simulink model "sin_osc_ver1"  (R2020a)
settings: Solver=ode14x  StartTime=0.0  StopTime=15  FixedStep=0.001  RelTol=1e-3
InitFcn:
  | init_param
StopFcn:
  | plot_out
values from neighbouring files (symbols this model uses):
  deltaT = 2*pi/(n*w)    (= 0.03125)    [init_param.m]
  k = 20    [init_param.m]
  r = 15 * 2*pi/360    (= 0.261799387799)    [init_param.m]
  sb = 1    [init_param.m]
  sf = 0    [init_param.m]
  t_sample = 0.001    [init_param.m]
  td = 0.01    [init_param.m]
  ts = deltaT    (= 0.03125)    [init_param.m]
  u0 = 0    [init_param.m]
  v0 = 0    [init_param.m]
  w = 4*pi    (= 12.5663706144)    [init_param.m]
libraries: dspsrcs4 x52
(part 1 of 2)
settings Model: Creator=QuangDuy  LastModifiedBy=QuangDuy

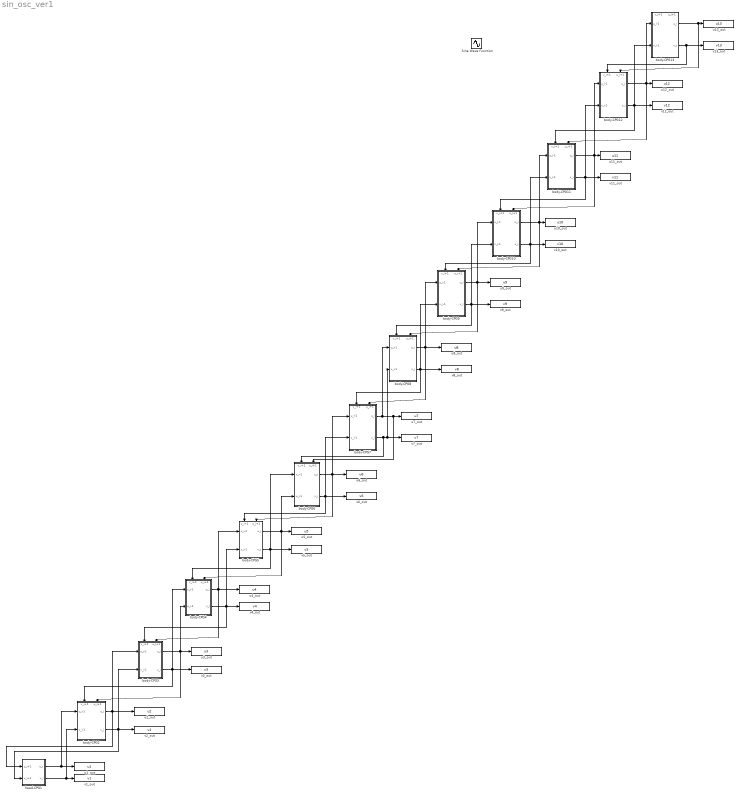
== system sin_osc_ver1 ==
  Sine Wave Function : Sin  TimeSource=Use external signal  SampleTime=0
  body-CPG10 : Subsystem
      settings: PortSchema="{\"entries\":[{\"content\":{\"sides\":[{\"content\":{\"connectorIds\":[\"In1\",\"In2\"]},\"type\":\"ConnectorPlacement.EquallySpacedRectSide\",\"uuid\":\"ffb19d8e-c609-407b-9735-0b1866f4cd92\"},{\"content\":{\"connectorIds\":[\"Out1\",\"Out2\"],\"side\":\"RIGHT\"},\"type\":\"ConnectorPlacement.EquallySpacedRectSide\",\"uuid\":\"e0704b2d-8456-48a5-a4d0-0d2061c5c352\"},{\"content\":{\"connectorIds\":[\"In3\",\"In4\"],\"side\":\"TOP\"},\"type\":\"ConnectorPlacement.EquallySpacedRectSide\",\"uuid\":\"2e0fb750-de55-423b-adb5-dbeaee2c2c2c\"}]},\"type\":\"ConnectorPlacement.EquallySpacedConnector\",\"uuid\":\"1ebf5890-2acb-4223-b38f-650141e84fec\"}],\"packageUris\":[\"http://schema.mathworks.com/mf0/Connector/19700101\"],\"version\":\"1.0\"}"
  body-CPG11 : Subsystem
      settings: PortSchema="{\"entries\":[{\"content\":{\"sides\":[{\"content\":{\"connectorIds\":[\"In1\",\"In2\"]},\"type\":\"ConnectorPlacement.EquallySpacedRectSide\",\"uuid\":\"ffb19d8e-c609-407b-9735-0b1866f4cd92\"},{\"content\":{\"connectorIds\":[\"Out1\",\"Out2\"],\"side\":\"RIGHT\"},\"type\":\"ConnectorPlacement.EquallySpacedRectSide\",\"uuid\":\"e0704b2d-8456-48a5-a4d0-0d2061c5c352\"},{\"content\":{\"connectorIds\":[\"In3\",\"In4\"],\"side\":\"TOP\"},\"type\":\"ConnectorPlacement.EquallySpacedRectSide\",\"uuid\":\"2e0fb750-de55-423b-adb5-dbeaee2c2c2c\"}]},\"type\":\"ConnectorPlacement.EquallySpacedConnector\",\"uuid\":\"1ebf5890-2acb-4223-b38f-650141e84fec\"}],\"packageUris\":[\"http://schema.mathworks.com/mf0/Connector/19700101\"],\"version\":\"1.0\"}"
  body-CPG12 : Subsystem
      settings: PortSchema="{\"entries\":[{\"content\":{\"sides\":[{\"content\":{\"connectorIds\":[\"In1\",\"In2\"]},\"type\":\"ConnectorPlacement.EquallySpacedRectSide\",\"uuid\":\"ffb19d8e-c609-407b-9735-0b1866f4cd92\"},{\"content\":{\"connectorIds\":[\"Out1\",\"Out2\"],\"side\":\"RIGHT\"},\"type\":\"ConnectorPlacement.EquallySpacedRectSide\",\"uuid\":\"e0704b2d-8456-48a5-a4d0-0d2061c5c352\"},{\"content\":{\"connectorIds\":[\"In3\",\"In4\"],\"side\":\"TOP\"},\"type\":\"ConnectorPlacement.EquallySpacedRectSide\",\"uuid\":\"2e0fb750-de55-423b-adb5-dbeaee2c2c2c\"}]},\"type\":\"ConnectorPlacement.EquallySpacedConnector\",\"uuid\":\"1ebf5890-2acb-4223-b38f-650141e84fec\"}],\"packageUris\":[\"http://schema.mathworks.com/mf0/Connector/19700101\"],\"version\":\"1.0\"}"
  body-CPG13 : Subsystem
      settings: PortSchema="{\"entries\":[{\"content\":{\"sides\":[{\"content\":{\"connectorIds\":[\"In1\",\"In2\"]},\"type\":\"ConnectorPlacement.EquallySpacedRectSide\",\"uuid\":\"ffb19d8e-c609-407b-9735-0b1866f4cd92\"},{\"content\":{\"connectorIds\":[\"Out1\",\"Out2\"],\"side\":\"RIGHT\"},\"type\":\"ConnectorPlacement.EquallySpacedRectSide\",\"uuid\":\"e0704b2d-8456-48a5-a4d0-0d2061c5c352\"},{\"content\":{\"connectorIds\":[\"In3\",\"In4\"],\"side\":\"TOP\"},\"type\":\"ConnectorPlacement.EquallySpacedRectSide\",\"uuid\":\"2e0fb750-de55-423b-adb5-dbeaee2c2c2c\"}]},\"type\":\"ConnectorPlacement.EquallySpacedConnector\",\"uuid\":\"1ebf5890-2acb-4223-b38f-650141e84fec\"}],\"packageUris\":[\"http://schema.mathworks.com/mf0/Connector/19700101\"],\"version\":\"1.0\"}"
  body-CPG2 : Subsystem
      settings: PortSchema="{\"entries\":[{\"content\":{\"sides\":[{\"content\":{\"connectorIds\":[\"In1\",\"In2\"]},\"type\":\"ConnectorPlacement.EquallySpacedRectSide\",\"uuid\":\"ffb19d8e-c609-407b-9735-0b1866f4cd92\"},{\"content\":{\"connectorIds\":[\"Out1\",\"Out2\"],\"side\":\"RIGHT\"},\"type\":\"ConnectorPlacement.EquallySpacedRectSide\",\"uuid\":\"e0704b2d-8456-48a5-a4d0-0d2061c5c352\"},{\"content\":{\"connectorIds\":[\"In3\",\"In4\"],\"side\":\"TOP\"},\"type\":\"ConnectorPlacement.EquallySpacedRectSide\",\"uuid\":\"2e0fb750-de55-423b-adb5-dbeaee2c2c2c\"}]},\"type\":\"ConnectorPlacement.EquallySpacedConnector\",\"uuid\":\"1ebf5890-2acb-4223-b38f-650141e84fec\"}],\"packageUris\":[\"http://schema.mathworks.com/mf0/Connector/19700101\"],\"version\":\"1.0\"}"
  body-CPG3 : Subsystem
      settings: PortSchema="{\"entries\":[{\"content\":{\"sides\":[{\"content\":{\"connectorIds\":[\"In1\",\"In2\"]},\"type\":\"ConnectorPlacement.EquallySpacedRectSide\",\"uuid\":\"ffb19d8e-c609-407b-9735-0b1866f4cd92\"},{\"content\":{\"connectorIds\":[\"Out1\",\"Out2\"],\"side\":\"RIGHT\"},\"type\":\"ConnectorPlacement.EquallySpacedRectSide\",\"uuid\":\"e0704b2d-8456-48a5-a4d0-0d2061c5c352\"},{\"content\":{\"connectorIds\":[\"In3\",\"In4\"],\"side\":\"TOP\"},\"type\":\"ConnectorPlacement.EquallySpacedRectSide\",\"uuid\":\"2e0fb750-de55-423b-adb5-dbeaee2c2c2c\"}]},\"type\":\"ConnectorPlacement.EquallySpacedConnector\",\"uuid\":\"1ebf5890-2acb-4223-b38f-650141e84fec\"}],\"packageUris\":[\"http://schema.mathworks.com/mf0/Connector/19700101\"],\"version\":\"1.0\"}"
  body-CPG4 : Subsystem
      settings: PortSchema="{\"entries\":[{\"content\":{\"sides\":[{\"content\":{\"connectorIds\":[\"In1\",\"In2\"]},\"type\":\"ConnectorPlacement.EquallySpacedRectSide\",\"uuid\":\"ffb19d8e-c609-407b-9735-0b1866f4cd92\"},{\"content\":{\"connectorIds\":[\"Out1\",\"Out2\"],\"side\":\"RIGHT\"},\"type\":\"ConnectorPlacement.EquallySpacedRectSide\",\"uuid\":\"e0704b2d-8456-48a5-a4d0-0d2061c5c352\"},{\"content\":{\"connectorIds\":[\"In3\",\"In4\"],\"side\":\"TOP\"},\"type\":\"ConnectorPlacement.EquallySpacedRectSide\",\"uuid\":\"2e0fb750-de55-423b-adb5-dbeaee2c2c2c\"}]},\"type\":\"ConnectorPlacement.EquallySpacedConnector\",\"uuid\":\"1ebf5890-2acb-4223-b38f-650141e84fec\"}],\"packageUris\":[\"http://schema.mathworks.com/mf0/Connector/19700101\"],\"version\":\"1.0\"}"
  body-CPG5 : Subsystem
      settings: PortSchema="{\"entries\":[{\"content\":{\"sides\":[{\"content\":{\"connectorIds\":[\"In1\",\"In2\"]},\"type\":\"ConnectorPlacement.EquallySpacedRectSide\",\"uuid\":\"ffb19d8e-c609-407b-9735-0b1866f4cd92\"},{\"content\":{\"connectorIds\":[\"Out1\",\"Out2\"],\"side\":\"RIGHT\"},\"type\":\"ConnectorPlacement.EquallySpacedRectSide\",\"uuid\":\"e0704b2d-8456-48a5-a4d0-0d2061c5c352\"},{\"content\":{\"connectorIds\":[\"In3\",\"In4\"],\"side\":\"TOP\"},\"type\":\"ConnectorPlacement.EquallySpacedRectSide\",\"uuid\":\"2e0fb750-de55-423b-adb5-dbeaee2c2c2c\"}]},\"type\":\"ConnectorPlacement.EquallySpacedConnector\",\"uuid\":\"1ebf5890-2acb-4223-b38f-650141e84fec\"}],\"packageUris\":[\"http://schema.mathworks.com/mf0/Connector/19700101\"],\"version\":\"1.0\"}"
  body-CPG6 : Subsystem
      settings: PortSchema="{\"entries\":[{\"content\":{\"sides\":[{\"content\":{\"connectorIds\":[\"In1\",\"In2\"]},\"type\":\"ConnectorPlacement.EquallySpacedRectSide\",\"uuid\":\"ffb19d8e-c609-407b-9735-0b1866f4cd92\"},{\"content\":{\"connectorIds\":[\"Out1\",\"Out2\"],\"side\":\"RIGHT\"},\"type\":\"ConnectorPlacement.EquallySpacedRectSide\",\"uuid\":\"e0704b2d-8456-48a5-a4d0-0d2061c5c352\"},{\"content\":{\"connectorIds\":[\"In3\",\"In4\"],\"side\":\"TOP\"},\"type\":\"ConnectorPlacement.EquallySpacedRectSide\",\"uuid\":\"2e0fb750-de55-423b-adb5-dbeaee2c2c2c\"}]},\"type\":\"ConnectorPlacement.EquallySpacedConnector\",\"uuid\":\"1ebf5890-2acb-4223-b38f-650141e84fec\"}],\"packageUris\":[\"http://schema.mathworks.com/mf0/Connector/19700101\"],\"version\":\"1.0\"}"
  body-CPG7 : Subsystem
      settings: PortSchema="{\"entries\":[{\"content\":{\"sides\":[{\"content\":{\"connectorIds\":[\"In1\",\"In2\"]},\"type\":\"ConnectorPlacement.EquallySpacedRectSide\",\"uuid\":\"ffb19d8e-c609-407b-9735-0b1866f4cd92\"},{\"content\":{\"connectorIds\":[\"Out1\",\"Out2\"],\"side\":\"RIGHT\"},\"type\":\"ConnectorPlacement.EquallySpacedRectSide\",\"uuid\":\"e0704b2d-8456-48a5-a4d0-0d2061c5c352\"},{\"content\":{\"connectorIds\":[\"In3\",\"In4\"],\"side\":\"TOP\"},\"type\":\"ConnectorPlacement.EquallySpacedRectSide\",\"uuid\":\"2e0fb750-de55-423b-adb5-dbeaee2c2c2c\"}]},\"type\":\"ConnectorPlacement.EquallySpacedConnector\",\"uuid\":\"1ebf5890-2acb-4223-b38f-650141e84fec\"}],\"packageUris\":[\"http://schema.mathworks.com/mf0/Connector/19700101\"],\"version\":\"1.0\"}"
  body-CPG8 : Subsystem
      settings: PortSchema="{\"entries\":[{\"content\":{\"sides\":[{\"content\":{\"connectorIds\":[\"In1\",\"In2\"]},\"type\":\"ConnectorPlacement.EquallySpacedRectSide\",\"uuid\":\"ffb19d8e-c609-407b-9735-0b1866f4cd92\"},{\"content\":{\"connectorIds\":[\"Out1\",\"Out2\"],\"side\":\"RIGHT\"},\"type\":\"ConnectorPlacement.EquallySpacedRectSide\",\"uuid\":\"e0704b2d-8456-48a5-a4d0-0d2061c5c352\"},{\"content\":{\"connectorIds\":[\"In3\",\"In4\"],\"side\":\"TOP\"},\"type\":\"ConnectorPlacement.EquallySpacedRectSide\",\"uuid\":\"2e0fb750-de55-423b-adb5-dbeaee2c2c2c\"}]},\"type\":\"ConnectorPlacement.EquallySpacedConnector\",\"uuid\":\"1ebf5890-2acb-4223-b38f-650141e84fec\"}],\"packageUris\":[\"http://schema.mathworks.com/mf0/Connector/19700101\"],\"version\":\"1.0\"}"
  body-CPG9 : Subsystem
      settings: PortSchema="{\"entries\":[{\"content\":{\"sides\":[{\"content\":{\"connectorIds\":[\"In1\",\"In2\"]},\"type\":\"ConnectorPlacement.EquallySpacedRectSide\",\"uuid\":\"ffb19d8e-c609-407b-9735-0b1866f4cd92\"},{\"content\":{\"connectorIds\":[\"Out1\",\"Out2\"],\"side\":\"RIGHT\"},\"type\":\"ConnectorPlacement.EquallySpacedRectSide\",\"uuid\":\"e0704b2d-8456-48a5-a4d0-0d2061c5c352\"},{\"content\":{\"connectorIds\":[\"In3\",\"In4\"],\"side\":\"TOP\"},\"type\":\"ConnectorPlacement.EquallySpacedRectSide\",\"uuid\":\"2e0fb750-de55-423b-adb5-dbeaee2c2c2c\"}]},\"type\":\"ConnectorPlacement.EquallySpacedConnector\",\"uuid\":\"1ebf5890-2acb-4223-b38f-650141e84fec\"}],\"packageUris\":[\"http://schema.mathworks.com/mf0/Connector/19700101\"],\"version\":\"1.0\"}"
  head-CPG1 : Subsystem
  u10_out : ToWorkspace  VariableName=u10  SampleTime=-1
  u11_out : ToWorkspace  VariableName=u11  SampleTime=-1
  u12_out : ToWorkspace  VariableName=u12  SampleTime=-1
  u13_out : ToWorkspace  VariableName=u13  SampleTime=-1
  u1_out : ToWorkspace  VariableName=u1  SampleTime=-1
  u2_out : ToWorkspace  VariableName=u2  SampleTime=-1
  u3_out : ToWorkspace  VariableName=u3  SampleTime=-1
  u4_out : ToWorkspace  VariableName=u4  SampleTime=-1
  u5_out : ToWorkspace  VariableName=u5  SampleTime=-1
  u6_out : ToWorkspace  VariableName=u6  SampleTime=-1
  u7_out : ToWorkspace  VariableName=u7  SampleTime=-1
  u8_out : ToWorkspace  VariableName=u8  SampleTime=-1
  u9_out : ToWorkspace  VariableName=u9  SampleTime=-1
  v10_out : ToWorkspace  VariableName=v10  SampleTime=-1
  v11_out : ToWorkspace  VariableName=v11  SampleTime=-1
  v12_out : ToWorkspace  VariableName=v12  SampleTime=-1
  v13_out : ToWorkspace  VariableName=v13  SampleTime=-1
  v1_out : ToWorkspace  VariableName=v1  SampleTime=-1
  v2_out : ToWorkspace  VariableName=v2  SampleTime=-1
  v3_out : ToWorkspace  VariableName=v3  SampleTime=-1
  v4_out : ToWorkspace  VariableName=v4  SampleTime=-1
  v5_out : ToWorkspace  VariableName=v5  SampleTime=-1
  v6_out : ToWorkspace  VariableName=v6  SampleTime=-1
  v7_out : ToWorkspace  VariableName=v7  SampleTime=-1
  v8_out : ToWorkspace  VariableName=v8  SampleTime=-1
  v9_out : ToWorkspace  VariableName=v9  SampleTime=-1
  wires:
  head-CPG1/1(u_i) -> body-CPG2/1(u_i-1), u1_out/1
  head-CPG1/2(v_i) -> body-CPG2/2(v_i-1), v1_out/1
  body-CPG2/2(v_i) -> head-CPG1/2(v_i+1), body-CPG3/2(v_i-1), v2_out/1
  body-CPG2/1(u_i) -> u2_out/1, head-CPG1/1(u_i+1), body-CPG3/1(u_i-1)
  body-CPG3/1(u_i) -> body-CPG4/2(u_i-1), u3_out/1, body-CPG2/4(u_i+1)
  body-CPG3/2(v_i) -> body-CPG2/3(v_i+1), body-CPG4/1(v_i-1), v3_out/1
  body-CPG4/1(u_i) -> body-CPG5/1(u_i-1), u4_out/1, body-CPG3/4(u_i+1)
  body-CPG4/2(v_i) -> body-CPG5/2(v_i-1), v4_out/1, body-CPG3/3(v_i+1)
  body-CPG5/2(v_i) -> body-CPG6/1(v_i-1), v5_out/1, body-CPG4/3(v_i+1)
  body-CPG5/1(u_i) -> body-CPG6/2(u_i-1), u5_out/1, body-CPG4/4(u_i+1)
  body-CPG6/1(u_i) -> body-CPG7/1(u_i-1), u6_out/1, body-CPG5/4(u_i+1)
  body-CPG6/2(v_i) -> body-CPG7/2(v_i-1), body-CPG5/3(v_i+1), v6_out/1
  body-CPG7/1(u_i) -> body-CPG8/1(u_i-1), body-CPG6/4(u_i+1), u7_out/1
  body-CPG7/2(v_i) -> body-CPG6/3(v_i+1), body-CPG8/2(v_i-1), v7_out/1
  body-CPG8/2(v_i) -> body-CPG9/2(v_i-1), v8_out/1, body-CPG7/3(v_i+1)
  body-CPG8/1(u_i) -> body-CPG9/1(u_i-1), body-CPG7/4(u_i+1), u8_out/1
  body-CPG9/2(v_i) -> body-CPG10/2(v_i-1), v9_out/1, body-CPG8/3(v_i+1)
  body-CPG9/1(u_i) -> body-CPG10/1(u_i-1), u9_out/1, body-CPG8/4(u_i+1)
  body-CPG10/2(v_i) -> body-CPG11/2(v_i-1), body-CPG9/3(v_i+1), v10_out/1
  body-CPG10/1(u_i) -> body-CPG9/4(u_i+1), body-CPG11/1(u_i-1), u10_out/1
  body-CPG11/2(v_i) -> body-CPG12/2(v_i-1), body-CPG10/3(v_i+1), v11_out/1
  body-CPG11/1(u_i) -> body-CPG10/4(u_i+1), body-CPG12/1(u_i-1), u11_out/1
  body-CPG12/2(v_i) -> body-CPG13/2(v_i-1), v12_out/1, body-CPG11/3(v_i+1)
  body-CPG12/1(u_i) -> body-CPG13/1(u_i-1), body-CPG11/4(u_i+1), u12_out/1
  body-CPG13/2(v_i) -> body-CPG12/3(v_i+1), v13_out/1
  body-CPG13/1(u_i) -> body-CPG12/4(u_i+1), u13_out/1

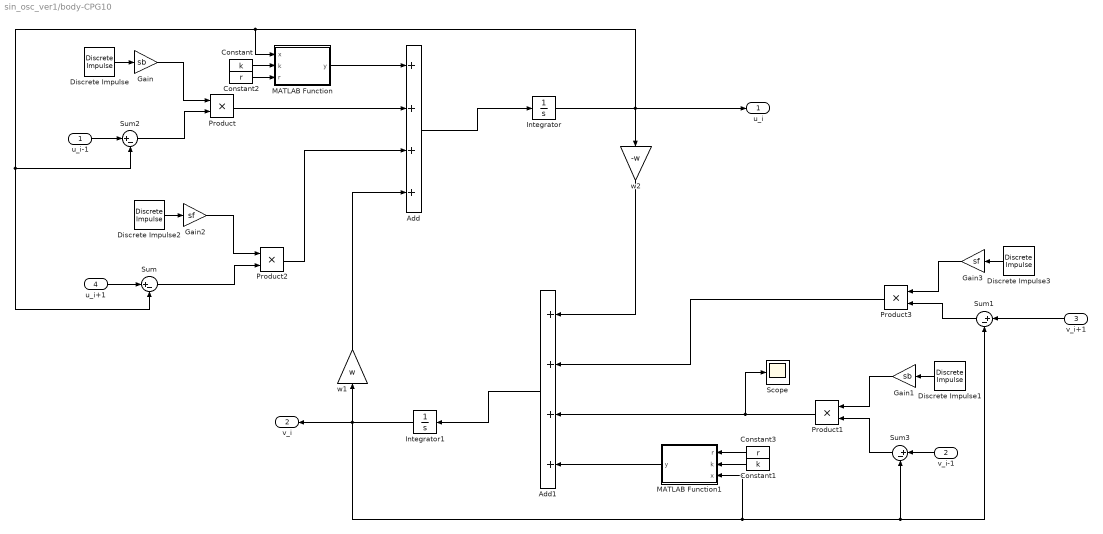
== system sin_osc_ver1/body-CPG10 ==
  u_i-1 : Inport
  v_i-1 : Inport  Port=2
  v_i+1 : Inport  Port=3
  u_i+1 : Inport  Port=4
  Add : Sum  Inputs=++++
  Add1 : Sum  Inputs=++++
  Constant : Constant  Value=k
  Constant1 : Constant  Value=k
  Constant2 : Constant  Value=r
  Constant3 : Constant  Value=r
  Discrete Impulse : dspsrcs4/Discrete  Impulse  Delay=round(10*deltaT/t_sample)+1  SampleTime=t_sample  FrameSample=1  OutputFrames=off  dataType=double  isSigned=on  wordLen=16  udDataType=sfix(16)  fracBitsMode=Best precision  numFracBits=15  OutDataTypeStr=double  LastOutDataTypeStr=double
  Discrete Impulse1 : dspsrcs4/Discrete  Impulse  Delay=round(10*deltaT/t_sample)  SampleTime=t_sample  FrameSample=1  OutputFrames=off  dataType=double  isSigned=on  wordLen=16  udDataType=sfix(16)  fracBitsMode=Best precision  numFracBits=15  OutDataTypeStr=double  LastOutDataTypeStr=double
  Discrete Impulse2 : dspsrcs4/Discrete  Impulse  Delay=round(10*deltaT/t_sample)+1  SampleTime=t_sample  FrameSample=1  OutputFrames=off  dataType=double  isSigned=on  wordLen=16  udDataType=sfix(16)  fracBitsMode=Best precision  numFracBits=15  OutDataTypeStr=double  LastOutDataTypeStr=double
  Discrete Impulse3 : dspsrcs4/Discrete  Impulse  Delay=round(10*deltaT/t_sample)  SampleTime=t_sample  FrameSample=1  OutputFrames=off  dataType=double  isSigned=on  wordLen=16  udDataType=sfix(16)  fracBitsMode=Best precision  numFracBits=15  OutDataTypeStr=double  LastOutDataTypeStr=double
  Gain : Gain  Gain=sb
  Gain1 : Gain  Gain=sb
  Gain2 : Gain  Gain=sf
  Gain3 : Gain  Gain=sf
  Integrator : Integrator  InitialCondition=u0
  Integrator1 : Integrator  InitialCondition=v0
  MATLAB Function : MATLAB Function  TreatAsAtomicUnit=on
  MATLAB Function1 : MATLAB Function  TreatAsAtomicUnit=on
  Product{,1..3} (4 alike) : Product
  Scope : Scope
  Sum{,1..3} (4 alike) : Sum  Inputs=|+-
  w1 : Gain  Gain=w
  w2 : Gain  Gain=-w
  u_i : Outport
  v_i : Outport  Port=2
  wires:
  Product2/1 -> Add/3
  Gain3/1 -> Product3/1
  w2/1 -> Add1/1
  Discrete Impulse1/1 -> Gain1/1
  Gain1/1 -> Product1/1
  Discrete Impulse/1 -> Gain/1
  Constant/1 -> MATLAB Function/2(k)
  Sum2/1 -> Product/2
  Add1/1 -> Integrator1/1
  Product1/1 -> Add1/3, Scope/1
  MATLAB Function/1(y) -> Add/1
  Discrete Impulse3/1 -> Gain3/1
  Product/1 -> Add/2
  Sum3/1 -> Product1/2
  Constant1/1 -> MATLAB Function1/2(k)
  w1/1 -> Add/4
  Integrator1/1 -> v_i/1, Sum3/2, Sum1/2, MATLAB Function1/3(x), w1/1
  Gain/1 -> Product/1
  Constant3/1 -> MATLAB Function1/1(r)
  Add/1 -> Integrator/1
  v_i+1/1 -> Sum1/1
  Sum/1 -> Product2/2
  Gain2/1 -> Product2/1
  Discrete Impulse2/1 -> Gain2/1
  Product3/1 -> Add1/2
  MATLAB Function1/1(y) -> Add1/4
  Constant2/1 -> MATLAB Function/3(r)
  u_i+1/1 -> Sum/1
  Sum1/1 -> Product3/2
  Integrator/1 -> u_i/1, Sum2/2, Sum/2, MATLAB Function/1(x), w2/1
  u_i-1/1 -> Sum2/1
  v_i-1/1 -> Sum3/1

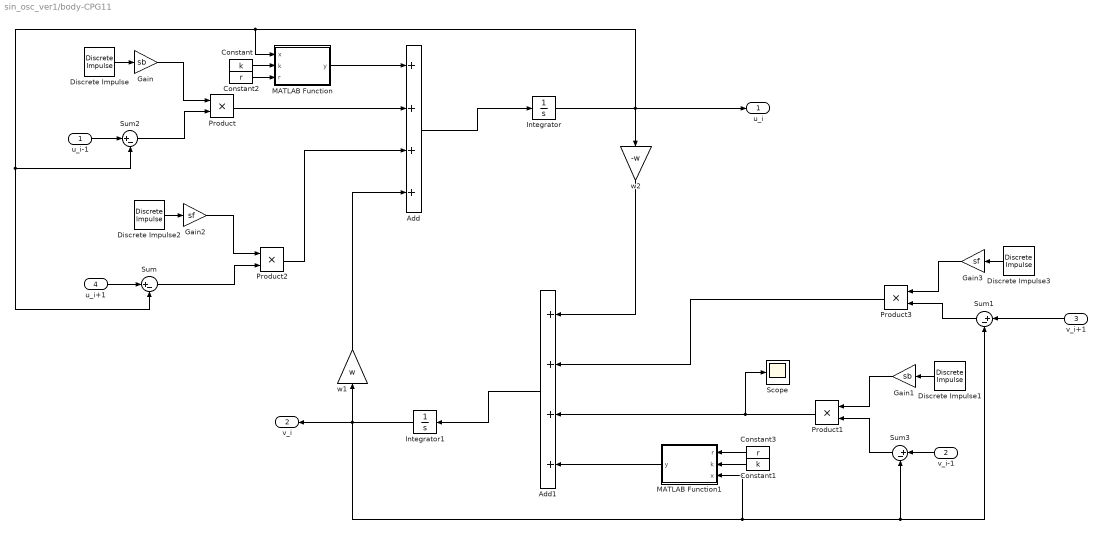
== system sin_osc_ver1/body-CPG11 ==
  u_i-1 : Inport
  v_i-1 : Inport  Port=2
  v_i+1 : Inport  Port=3
  u_i+1 : Inport  Port=4
  Add : Sum  Inputs=++++
  Add1 : Sum  Inputs=++++
  Constant : Constant  Value=k
  Constant1 : Constant  Value=k
  Constant2 : Constant  Value=r
  Constant3 : Constant  Value=r
  Discrete Impulse : dspsrcs4/Discrete  Impulse  Delay=round(11*deltaT/t_sample)+1  SampleTime=t_sample  FrameSample=1  OutputFrames=off  dataType=double  isSigned=on  wordLen=16  udDataType=sfix(16)  fracBitsMode=Best precision  numFracBits=15  OutDataTypeStr=double  LastOutDataTypeStr=double
  Discrete Impulse1 : dspsrcs4/Discrete  Impulse  Delay=round(11*deltaT/t_sample)  SampleTime=t_sample  FrameSample=1  OutputFrames=off  dataType=double  isSigned=on  wordLen=16  udDataType=sfix(16)  fracBitsMode=Best precision  numFracBits=15  OutDataTypeStr=double  LastOutDataTypeStr=double
  Discrete Impulse2 : dspsrcs4/Discrete  Impulse  Delay=round(11*deltaT/t_sample)+1  SampleTime=t_sample  FrameSample=1  OutputFrames=off  dataType=double  isSigned=on  wordLen=16  udDataType=sfix(16)  fracBitsMode=Best precision  numFracBits=15  OutDataTypeStr=double  LastOutDataTypeStr=double
  Discrete Impulse3 : dspsrcs4/Discrete  Impulse  Delay=round(11*deltaT/t_sample)  SampleTime=t_sample  FrameSample=1  OutputFrames=off  dataType=double  isSigned=on  wordLen=16  udDataType=sfix(16)  fracBitsMode=Best precision  numFracBits=15  OutDataTypeStr=double  LastOutDataTypeStr=double
  Gain : Gain  Gain=sb
  Gain1 : Gain  Gain=sb
  Gain2 : Gain  Gain=sf
  Gain3 : Gain  Gain=sf
  Integrator : Integrator  InitialCondition=u0
  Integrator1 : Integrator  InitialCondition=v0
  MATLAB Function : MATLAB Function  TreatAsAtomicUnit=on
  MATLAB Function1 : MATLAB Function  TreatAsAtomicUnit=on
  Product{,1..3} (4 alike) : Product
  Scope : Scope
  Sum{,1..3} (4 alike) : Sum  Inputs=|+-
  w1 : Gain  Gain=w
  w2 : Gain  Gain=-w
  u_i : Outport
  v_i : Outport  Port=2
  wires:
  Product2/1 -> Add/3
  Gain3/1 -> Product3/1
  w2/1 -> Add1/1
  Discrete Impulse1/1 -> Gain1/1
  Gain1/1 -> Product1/1
  Discrete Impulse/1 -> Gain/1
  Constant/1 -> MATLAB Function/2(k)
  Sum2/1 -> Product/2
  Add1/1 -> Integrator1/1
  Product1/1 -> Add1/3, Scope/1
  MATLAB Function/1(y) -> Add/1
  Discrete Impulse3/1 -> Gain3/1
  Product/1 -> Add/2
  Sum3/1 -> Product1/2
  Constant1/1 -> MATLAB Function1/2(k)
  w1/1 -> Add/4
  Integrator1/1 -> v_i/1, Sum3/2, Sum1/2, MATLAB Function1/3(x), w1/1
  Gain/1 -> Product/1
  Constant3/1 -> MATLAB Function1/1(r)
  Add/1 -> Integrator/1
  v_i+1/1 -> Sum1/1
  Sum/1 -> Product2/2
  Gain2/1 -> Product2/1
  Discrete Impulse2/1 -> Gain2/1
  Product3/1 -> Add1/2
  MATLAB Function1/1(y) -> Add1/4
  Constant2/1 -> MATLAB Function/3(r)
  u_i+1/1 -> Sum/1
  Sum1/1 -> Product3/2
  Integrator/1 -> u_i/1, Sum2/2, Sum/2, MATLAB Function/1(x), w2/1
  u_i-1/1 -> Sum2/1
  v_i-1/1 -> Sum3/1

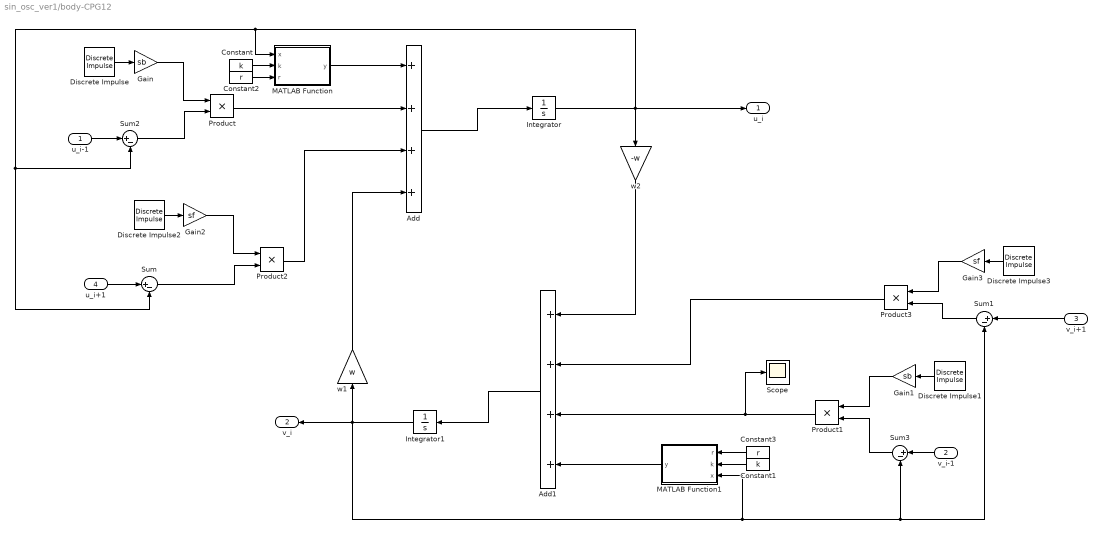
== system sin_osc_ver1/body-CPG12 ==
  u_i-1 : Inport
  v_i-1 : Inport  Port=2
  v_i+1 : Inport  Port=3
  u_i+1 : Inport  Port=4
  Add : Sum  Inputs=++++
  Add1 : Sum  Inputs=++++
  Constant : Constant  Value=k
  Constant1 : Constant  Value=k
  Constant2 : Constant  Value=r
  Constant3 : Constant  Value=r
  Discrete Impulse : dspsrcs4/Discrete  Impulse  Delay=round(12*deltaT/t_sample)+1  SampleTime=t_sample  FrameSample=1  OutputFrames=off  dataType=double  isSigned=on  wordLen=16  udDataType=sfix(16)  fracBitsMode=Best precision  numFracBits=15  OutDataTypeStr=double  LastOutDataTypeStr=double
  Discrete Impulse1 : dspsrcs4/Discrete  Impulse  Delay=round(12*deltaT/t_sample)  SampleTime=t_sample  FrameSample=1  OutputFrames=off  dataType=double  isSigned=on  wordLen=16  udDataType=sfix(16)  fracBitsMode=Best precision  numFracBits=15  OutDataTypeStr=double  LastOutDataTypeStr=double
  Discrete Impulse2 : dspsrcs4/Discrete  Impulse  Delay=round(12*deltaT/t_sample)+1  SampleTime=t_sample  FrameSample=1  OutputFrames=off  dataType=double  isSigned=on  wordLen=16  udDataType=sfix(16)  fracBitsMode=Best precision  numFracBits=15  OutDataTypeStr=double  LastOutDataTypeStr=double
  Discrete Impulse3 : dspsrcs4/Discrete  Impulse  Delay=round(12*deltaT/t_sample)  SampleTime=t_sample  FrameSample=1  OutputFrames=off  dataType=double  isSigned=on  wordLen=16  udDataType=sfix(16)  fracBitsMode=Best precision  numFracBits=15  OutDataTypeStr=double  LastOutDataTypeStr=double
  Gain : Gain  Gain=sb
  Gain1 : Gain  Gain=sb
  Gain2 : Gain  Gain=sf
  Gain3 : Gain  Gain=sf
  Integrator : Integrator  InitialCondition=u0
  Integrator1 : Integrator  InitialCondition=v0
  MATLAB Function : MATLAB Function  TreatAsAtomicUnit=on
  MATLAB Function1 : MATLAB Function  TreatAsAtomicUnit=on
  Product{,1..3} (4 alike) : Product
  Scope : Scope
  Sum{,1..3} (4 alike) : Sum  Inputs=|+-
  w1 : Gain  Gain=w
  w2 : Gain  Gain=-w
  u_i : Outport
  v_i : Outport  Port=2
  wires:
  Product2/1 -> Add/3
  Gain3/1 -> Product3/1
  w2/1 -> Add1/1
  Discrete Impulse1/1 -> Gain1/1
  Gain1/1 -> Product1/1
  Discrete Impulse/1 -> Gain/1
  Constant/1 -> MATLAB Function/2(k)
  Sum2/1 -> Product/2
  Add1/1 -> Integrator1/1
  Product1/1 -> Add1/3, Scope/1
  MATLAB Function/1(y) -> Add/1
  Discrete Impulse3/1 -> Gain3/1
  Product/1 -> Add/2
  Sum3/1 -> Product1/2
  Constant1/1 -> MATLAB Function1/2(k)
  w1/1 -> Add/4
  Integrator1/1 -> v_i/1, Sum3/2, Sum1/2, MATLAB Function1/3(x), w1/1
  Gain/1 -> Product/1
  Constant3/1 -> MATLAB Function1/1(r)
  Add/1 -> Integrator/1
  v_i+1/1 -> Sum1/1
  Sum/1 -> Product2/2
  Gain2/1 -> Product2/1
  Discrete Impulse2/1 -> Gain2/1
  Product3/1 -> Add1/2
  MATLAB Function1/1(y) -> Add1/4
  Constant2/1 -> MATLAB Function/3(r)
  u_i+1/1 -> Sum/1
  Sum1/1 -> Product3/2
  Integrator/1 -> u_i/1, Sum2/2, Sum/2, MATLAB Function/1(x), w2/1
  u_i-1/1 -> Sum2/1
  v_i-1/1 -> Sum3/1

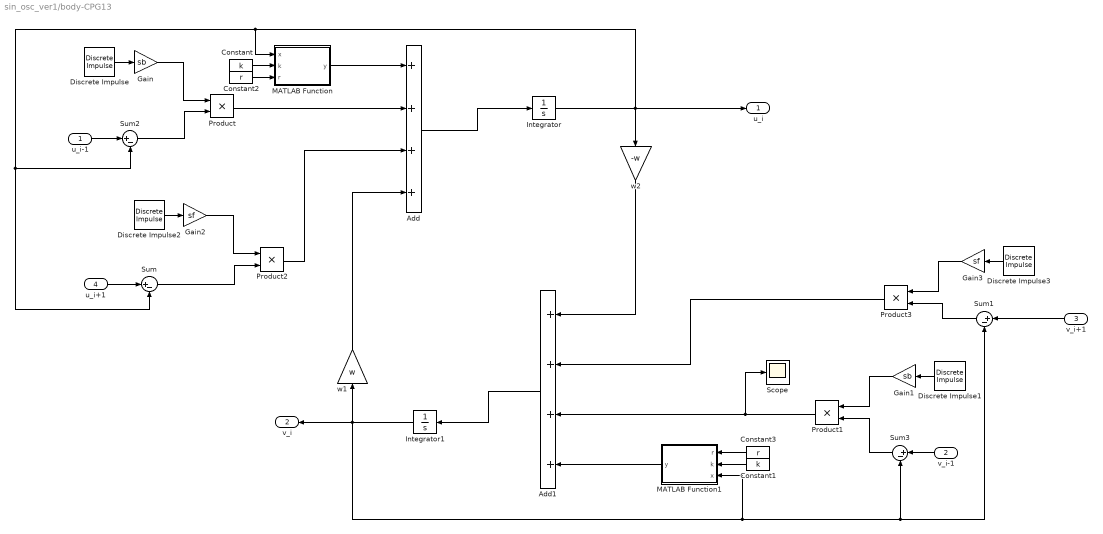
== system sin_osc_ver1/body-CPG13 ==
  u_i-1 : Inport
  v_i-1 : Inport  Port=2
  v_i+1 : Inport  Port=3
  u_i+1 : Inport  Port=4
  Add : Sum  Inputs=++++
  Add1 : Sum  Inputs=++++
  Constant : Constant  Value=k
  Constant1 : Constant  Value=k
  Constant2 : Constant  Value=r
  Constant3 : Constant  Value=r
  Discrete Impulse : dspsrcs4/Discrete  Impulse  Delay=round(13*deltaT/t_sample)+1  SampleTime=t_sample  FrameSample=1  OutputFrames=off  dataType=double  isSigned=on  wordLen=16  udDataType=sfix(16)  fracBitsMode=Best precision  numFracBits=15  OutDataTypeStr=double  LastOutDataTypeStr=double
  Discrete Impulse1 : dspsrcs4/Discrete  Impulse  Delay=round(13*deltaT/t_sample)  SampleTime=t_sample  FrameSample=1  OutputFrames=off  dataType=double  isSigned=on  wordLen=16  udDataType=sfix(16)  fracBitsMode=Best precision  numFracBits=15  OutDataTypeStr=double  LastOutDataTypeStr=double
  Discrete Impulse2 : dspsrcs4/Discrete  Impulse  Delay=round(13*deltaT/t_sample)+1  SampleTime=t_sample  FrameSample=1  OutputFrames=off  dataType=double  isSigned=on  wordLen=16  udDataType=sfix(16)  fracBitsMode=Best precision  numFracBits=15  OutDataTypeStr=double  LastOutDataTypeStr=double
  Discrete Impulse3 : dspsrcs4/Discrete  Impulse  Delay=round(13*deltaT/t_sample)  SampleTime=t_sample  FrameSample=1  OutputFrames=off  dataType=double  isSigned=on  wordLen=16  udDataType=sfix(16)  fracBitsMode=Best precision  numFracBits=15  OutDataTypeStr=double  LastOutDataTypeStr=double
  Gain : Gain  Gain=sb
  Gain1 : Gain  Gain=sb
  Gain2 : Gain  Gain=sf
  Gain3 : Gain  Gain=sf
  Integrator : Integrator  InitialCondition=u0
  Integrator1 : Integrator  InitialCondition=v0
  MATLAB Function : MATLAB Function  TreatAsAtomicUnit=on
  MATLAB Function1 : MATLAB Function  TreatAsAtomicUnit=on
  Product{,1..3} (4 alike) : Product
  Scope : Scope
  Sum{,1..3} (4 alike) : Sum  Inputs=|+-
  w1 : Gain  Gain=w
  w2 : Gain  Gain=-w
  u_i : Outport
  v_i : Outport  Port=2
  wires:
  Product2/1 -> Add/3
  Gain3/1 -> Product3/1
  w2/1 -> Add1/1
  Discrete Impulse1/1 -> Gain1/1
  Gain1/1 -> Product1/1
  Discrete Impulse/1 -> Gain/1
  Constant/1 -> MATLAB Function/2(k)
  Sum2/1 -> Product/2
  Add1/1 -> Integrator1/1
  Product1/1 -> Add1/3, Scope/1
  MATLAB Function/1(y) -> Add/1
  Discrete Impulse3/1 -> Gain3/1
  Product/1 -> Add/2
  Sum3/1 -> Product1/2
  Constant1/1 -> MATLAB Function1/2(k)
  w1/1 -> Add/4
  Integrator1/1 -> v_i/1, Sum3/2, Sum1/2, MATLAB Function1/3(x), w1/1
  Gain/1 -> Product/1
  Constant3/1 -> MATLAB Function1/1(r)
  Add/1 -> Integrator/1
  v_i+1/1 -> Sum1/1
  Sum/1 -> Product2/2
  Gain2/1 -> Product2/1
  Discrete Impulse2/1 -> Gain2/1
  Product3/1 -> Add1/2
  MATLAB Function1/1(y) -> Add1/4
  Constant2/1 -> MATLAB Function/3(r)
  u_i+1/1 -> Sum/1
  Sum1/1 -> Product3/2
  Integrator/1 -> u_i/1, Sum2/2, Sum/2, MATLAB Function/1(x), w2/1
  u_i-1/1 -> Sum2/1
  v_i-1/1 -> Sum3/1

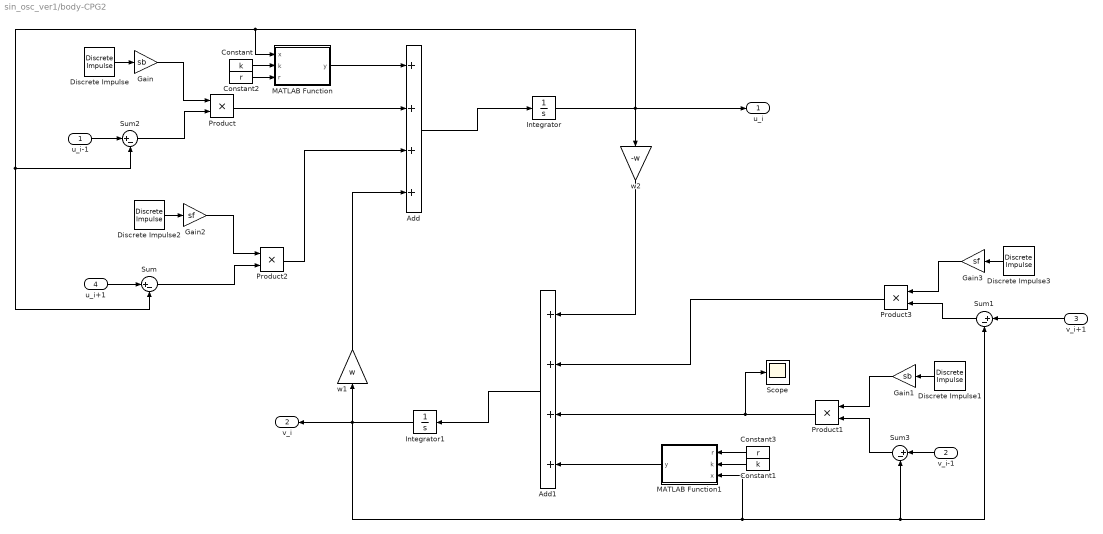
== system sin_osc_ver1/body-CPG2 ==
  u_i-1 : Inport
  v_i-1 : Inport  Port=2
  v_i+1 : Inport  Port=3
  u_i+1 : Inport  Port=4
  Add : Sum  Inputs=++++
  Add1 : Sum  Inputs=++++
  Constant : Constant  Value=k
  Constant1 : Constant  Value=k
  Constant2 : Constant  Value=r
  Constant3 : Constant  Value=r
  Discrete Impulse : dspsrcs4/Discrete  Impulse  Delay=round(2*deltaT/t_sample)+1  SampleTime=t_sample  FrameSample=1  OutputFrames=off  dataType=double  isSigned=on  wordLen=16  udDataType=sfix(16)  fracBitsMode=Best precision  numFracBits=15  OutDataTypeStr=double  LastOutDataTypeStr=double
  Discrete Impulse1 : dspsrcs4/Discrete  Impulse  Delay=round(2*deltaT/t_sample)  SampleTime=t_sample  FrameSample=1  OutputFrames=off  dataType=double  isSigned=on  wordLen=16  udDataType=sfix(16)  fracBitsMode=Best precision  numFracBits=15  OutDataTypeStr=double  LastOutDataTypeStr=double
  Discrete Impulse2 : dspsrcs4/Discrete  Impulse  Delay=round(2*deltaT/t_sample)+1  SampleTime=t_sample  FrameSample=1  OutputFrames=off  dataType=double  isSigned=on  wordLen=16  udDataType=sfix(16)  fracBitsMode=Best precision  numFracBits=15  OutDataTypeStr=double  LastOutDataTypeStr=double
  Discrete Impulse3 : dspsrcs4/Discrete  Impulse  Delay=round(2*deltaT/t_sample)  SampleTime=t_sample  FrameSample=1  OutputFrames=off  dataType=double  isSigned=on  wordLen=16  udDataType=sfix(16)  fracBitsMode=Best precision  numFracBits=15  OutDataTypeStr=double  LastOutDataTypeStr=double
  Gain : Gain  Gain=sb
  Gain1 : Gain  Gain=sb
  Gain2 : Gain  Gain=sf
  Gain3 : Gain  Gain=sf
  Integrator : Integrator  InitialCondition=u0
  Integrator1 : Integrator  InitialCondition=v0
  MATLAB Function : MATLAB Function  TreatAsAtomicUnit=on
  MATLAB Function1 : MATLAB Function  TreatAsAtomicUnit=on
  Product{,1..3} (4 alike) : Product
  Scope : Scope
  Sum{,1..3} (4 alike) : Sum  Inputs=|+-
  w1 : Gain  Gain=w
  w2 : Gain  Gain=-w
  u_i : Outport
  v_i : Outport  Port=2
  wires:
  Product2/1 -> Add/3
  Gain3/1 -> Product3/1
  w2/1 -> Add1/1
  Discrete Impulse1/1 -> Gain1/1
  Gain1/1 -> Product1/1
  Discrete Impulse/1 -> Gain/1
  Constant/1 -> MATLAB Function/2(k)
  Sum2/1 -> Product/2
  Add1/1 -> Integrator1/1
  Product1/1 -> Add1/3, Scope/1
  MATLAB Function/1(y) -> Add/1
  Discrete Impulse3/1 -> Gain3/1
  Product/1 -> Add/2
  Sum3/1 -> Product1/2
  Constant1/1 -> MATLAB Function1/2(k)
  w1/1 -> Add/4
  Integrator1/1 -> v_i/1, Sum3/2, Sum1/2, MATLAB Function1/3(x), w1/1
  Gain/1 -> Product/1
  Constant3/1 -> MATLAB Function1/1(r)
  Add/1 -> Integrator/1
  v_i+1/1 -> Sum1/1
  Sum/1 -> Product2/2
  Gain2/1 -> Product2/1
  Discrete Impulse2/1 -> Gain2/1
  Product3/1 -> Add1/2
  MATLAB Function1/1(y) -> Add1/4
  Constant2/1 -> MATLAB Function/3(r)
  u_i+1/1 -> Sum/1
  Sum1/1 -> Product3/2
  Integrator/1 -> u_i/1, Sum2/2, Sum/2, MATLAB Function/1(x), w2/1
  u_i-1/1 -> Sum2/1
  v_i-1/1 -> Sum3/1

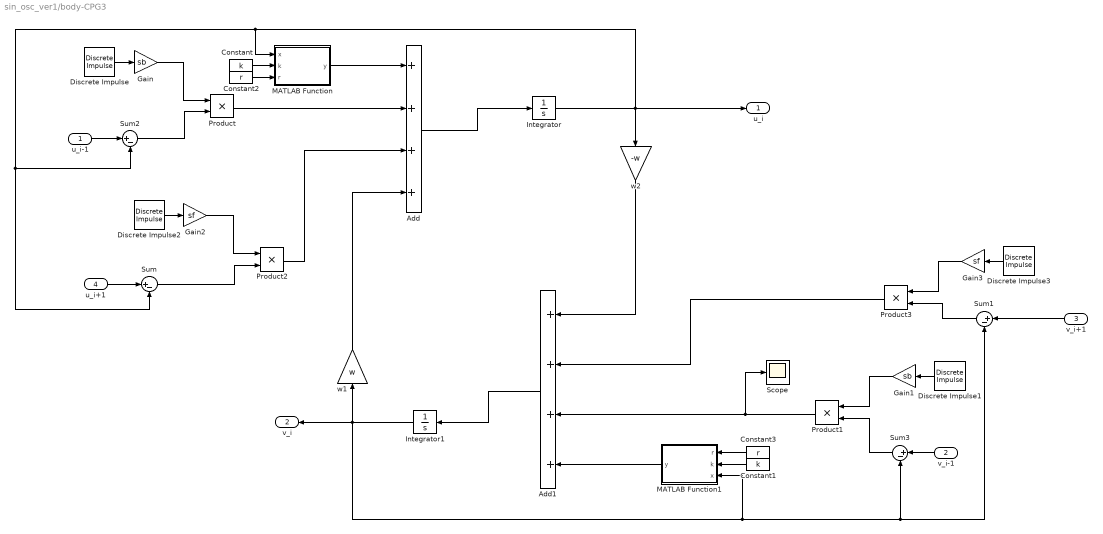
== system sin_osc_ver1/body-CPG3 ==
  u_i-1 : Inport
  v_i-1 : Inport  Port=2
  v_i+1 : Inport  Port=3
  u_i+1 : Inport  Port=4
  Add : Sum  Inputs=++++
  Add1 : Sum  Inputs=++++
  Constant : Constant  Value=k
  Constant1 : Constant  Value=k
  Constant2 : Constant  Value=r
  Constant3 : Constant  Value=r
  Discrete Impulse : dspsrcs4/Discrete  Impulse  Delay=round(3*deltaT/t_sample)+1  SampleTime=t_sample  FrameSample=1  OutputFrames=off  dataType=double  isSigned=on  wordLen=16  udDataType=sfix(16)  fracBitsMode=Best precision  numFracBits=15  OutDataTypeStr=double  LastOutDataTypeStr=double
  Discrete Impulse1 : dspsrcs4/Discrete  Impulse  Delay=round(3*deltaT/t_sample)  SampleTime=t_sample  FrameSample=1  OutputFrames=off  dataType=double  isSigned=on  wordLen=16  udDataType=sfix(16)  fracBitsMode=Best precision  numFracBits=15  OutDataTypeStr=double  LastOutDataTypeStr=double
  Discrete Impulse2 : dspsrcs4/Discrete  Impulse  Delay=round(3*deltaT/t_sample)+1  SampleTime=t_sample  FrameSample=1  OutputFrames=off  dataType=double  isSigned=on  wordLen=16  udDataType=sfix(16)  fracBitsMode=Best precision  numFracBits=15  OutDataTypeStr=double  LastOutDataTypeStr=double
  Discrete Impulse3 : dspsrcs4/Discrete  Impulse  Delay=round(3*deltaT/t_sample)  SampleTime=t_sample  FrameSample=1  OutputFrames=off  dataType=double  isSigned=on  wordLen=16  udDataType=sfix(16)  fracBitsMode=Best precision  numFracBits=15  OutDataTypeStr=double  LastOutDataTypeStr=double
  Gain : Gain  Gain=sb
  Gain1 : Gain  Gain=sb
  Gain2 : Gain  Gain=sf
  Gain3 : Gain  Gain=sf
  Integrator : Integrator  InitialCondition=u0
  Integrator1 : Integrator  InitialCondition=v0
  MATLAB Function : MATLAB Function  TreatAsAtomicUnit=on
  MATLAB Function1 : MATLAB Function  TreatAsAtomicUnit=on
  Product{,1..3} (4 alike) : Product
  Scope : Scope
  Sum{,1..3} (4 alike) : Sum  Inputs=|+-
  w1 : Gain  Gain=w
  w2 : Gain  Gain=-w
  u_i : Outport
  v_i : Outport  Port=2
  wires:
  Product2/1 -> Add/3
  Gain3/1 -> Product3/1
  w2/1 -> Add1/1
  Discrete Impulse1/1 -> Gain1/1
  Gain1/1 -> Product1/1
  Discrete Impulse/1 -> Gain/1
  Constant/1 -> MATLAB Function/2(k)
  Sum2/1 -> Product/2
  Add1/1 -> Integrator1/1
  Product1/1 -> Add1/3, Scope/1
  MATLAB Function/1(y) -> Add/1
  Discrete Impulse3/1 -> Gain3/1
  Product/1 -> Add/2
  Sum3/1 -> Product1/2
  Constant1/1 -> MATLAB Function1/2(k)
  w1/1 -> Add/4
  Integrator1/1 -> v_i/1, Sum3/2, Sum1/2, MATLAB Function1/3(x), w1/1
  Gain/1 -> Product/1
  Constant3/1 -> MATLAB Function1/1(r)
  Add/1 -> Integrator/1
  v_i+1/1 -> Sum1/1
  Sum/1 -> Product2/2
  Gain2/1 -> Product2/1
  Discrete Impulse2/1 -> Gain2/1
  Product3/1 -> Add1/2
  MATLAB Function1/1(y) -> Add1/4
  Constant2/1 -> MATLAB Function/3(r)
  u_i+1/1 -> Sum/1
  Sum1/1 -> Product3/2
  Integrator/1 -> u_i/1, Sum2/2, Sum/2, MATLAB Function/1(x), w2/1
  u_i-1/1 -> Sum2/1
  v_i-1/1 -> Sum3/1

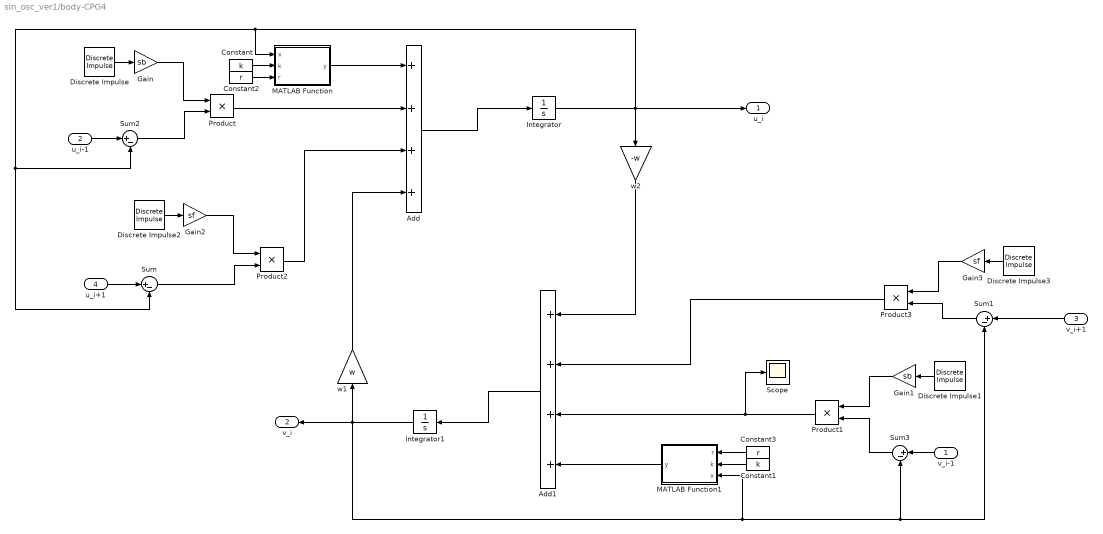
== system sin_osc_ver1/body-CPG4 ==
  v_i-1 : Inport
  u_i-1 : Inport  Port=2
  v_i+1 : Inport  Port=3
  u_i+1 : Inport  Port=4
  Add : Sum  Inputs=++++
  Add1 : Sum  Inputs=++++
  Constant : Constant  Value=k
  Constant1 : Constant  Value=k
  Constant2 : Constant  Value=r
  Constant3 : Constant  Value=r
  Discrete Impulse : dspsrcs4/Discrete  Impulse  Delay=round(4*deltaT/t_sample)+1  SampleTime=t_sample  FrameSample=1  OutputFrames=off  dataType=double  isSigned=on  wordLen=16  udDataType=sfix(16)  fracBitsMode=Best precision  numFracBits=15  OutDataTypeStr=double  LastOutDataTypeStr=double
  Discrete Impulse1 : dspsrcs4/Discrete  Impulse  Delay=round(4*deltaT/t_sample)  SampleTime=t_sample  FrameSample=1  OutputFrames=off  dataType=double  isSigned=on  wordLen=16  udDataType=sfix(16)  fracBitsMode=Best precision  numFracBits=15  OutDataTypeStr=double  LastOutDataTypeStr=double
  Discrete Impulse2 : dspsrcs4/Discrete  Impulse  Delay=round(4*deltaT/t_sample)+1  SampleTime=t_sample  FrameSample=1  OutputFrames=off  dataType=double  isSigned=on  wordLen=16  udDataType=sfix(16)  fracBitsMode=Best precision  numFracBits=15  OutDataTypeStr=double  LastOutDataTypeStr=double
  Discrete Impulse3 : dspsrcs4/Discrete  Impulse  Delay=round(4*deltaT/t_sample)  SampleTime=t_sample  FrameSample=1  OutputFrames=off  dataType=double  isSigned=on  wordLen=16  udDataType=sfix(16)  fracBitsMode=Best precision  numFracBits=15  OutDataTypeStr=double  LastOutDataTypeStr=double
  Gain : Gain  Gain=sb
  Gain1 : Gain  Gain=sb
  Gain2 : Gain  Gain=sf
  Gain3 : Gain  Gain=sf
  Integrator : Integrator  InitialCondition=u0
  Integrator1 : Integrator  InitialCondition=v0
  MATLAB Function : MATLAB Function  TreatAsAtomicUnit=on
  MATLAB Function1 : MATLAB Function  TreatAsAtomicUnit=on
  Product{,1..3} (4 alike) : Product
  Scope : Scope
  Sum{,1..3} (4 alike) : Sum  Inputs=|+-
  w1 : Gain  Gain=w
  w2 : Gain  Gain=-w
  u_i : Outport
  v_i : Outport  Port=2
  wires:
  Product2/1 -> Add/3
  Gain3/1 -> Product3/1
  w2/1 -> Add1/1
  Discrete Impulse1/1 -> Gain1/1
  Gain1/1 -> Product1/1
  Discrete Impulse/1 -> Gain/1
  Constant/1 -> MATLAB Function/2(k)
  Sum2/1 -> Product/2
  Add1/1 -> Integrator1/1
  Product1/1 -> Add1/3, Scope/1
  MATLAB Function/1(y) -> Add/1
  Discrete Impulse3/1 -> Gain3/1
  Product/1 -> Add/2
  Sum3/1 -> Product1/2
  Constant1/1 -> MATLAB Function1/2(k)
  w1/1 -> Add/4
  Integrator1/1 -> v_i/1, Sum3/2, Sum1/2, MATLAB Function1/3(x), w1/1
  Gain/1 -> Product/1
  Constant3/1 -> MATLAB Function1/1(r)
  Add/1 -> Integrator/1
  v_i+1/1 -> Sum1/1
  Sum/1 -> Product2/2
  Gain2/1 -> Product2/1
  Discrete Impulse2/1 -> Gain2/1
  Product3/1 -> Add1/2
  MATLAB Function1/1(y) -> Add1/4
  Constant2/1 -> MATLAB Function/3(r)
  u_i+1/1 -> Sum/1
  Sum1/1 -> Product3/2
  Integrator/1 -> u_i/1, Sum2/2, Sum/2, MATLAB Function/1(x), w2/1
  u_i-1/1 -> Sum2/1
  v_i-1/1 -> Sum3/1

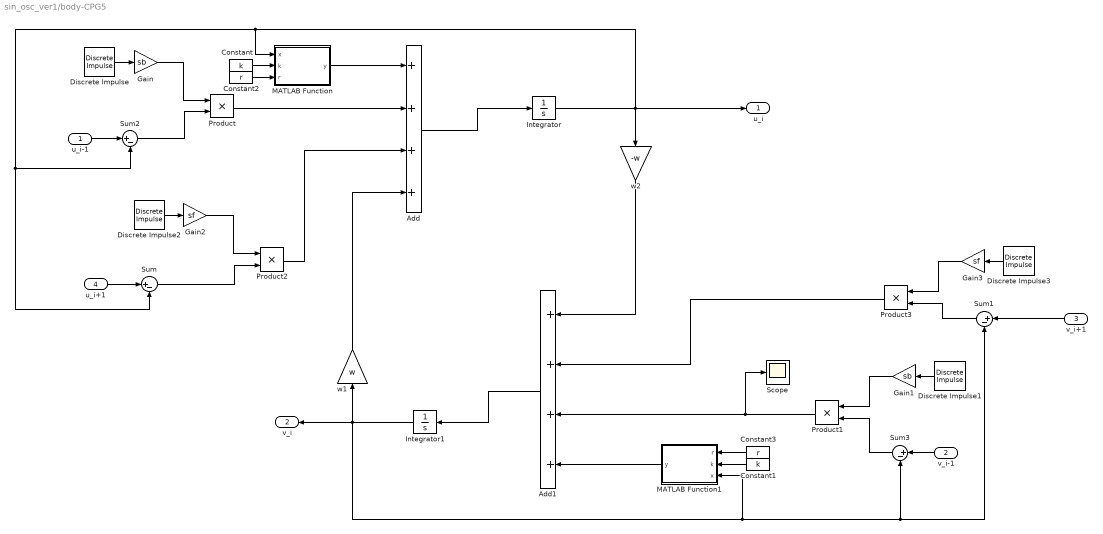
== system sin_osc_ver1/body-CPG5 ==
  u_i-1 : Inport
  v_i-1 : Inport  Port=2
  v_i+1 : Inport  Port=3
  u_i+1 : Inport  Port=4
  Add : Sum  Inputs=++++
  Add1 : Sum  Inputs=++++
  Constant : Constant  Value=k
  Constant1 : Constant  Value=k
  Constant2 : Constant  Value=r
  Constant3 : Constant  Value=r
  Discrete Impulse : dspsrcs4/Discrete  Impulse  Delay=round(5*deltaT/t_sample)+1  SampleTime=t_sample  FrameSample=1  OutputFrames=off  dataType=double  isSigned=on  wordLen=16  udDataType=sfix(16)  fracBitsMode=Best precision  numFracBits=15  OutDataTypeStr=double  LastOutDataTypeStr=double
  Discrete Impulse1 : dspsrcs4/Discrete  Impulse  Delay=round(5*deltaT/t_sample)  SampleTime=t_sample  FrameSample=1  OutputFrames=off  dataType=double  isSigned=on  wordLen=16  udDataType=sfix(16)  fracBitsMode=Best precision  numFracBits=15  OutDataTypeStr=double  LastOutDataTypeStr=double
  Discrete Impulse2 : dspsrcs4/Discrete  Impulse  Delay=round(5*deltaT/t_sample)+1  SampleTime=t_sample  FrameSample=1  OutputFrames=off  dataType=double  isSigned=on  wordLen=16  udDataType=sfix(16)  fracBitsMode=Best precision  numFracBits=15  OutDataTypeStr=double  LastOutDataTypeStr=double
  Discrete Impulse3 : dspsrcs4/Discrete  Impulse  Delay=round(5*deltaT/t_sample)  SampleTime=t_sample  FrameSample=1  OutputFrames=off  dataType=double  isSigned=on  wordLen=16  udDataType=sfix(16)  fracBitsMode=Best precision  numFracBits=15  OutDataTypeStr=double  LastOutDataTypeStr=double
  Gain : Gain  Gain=sb
  Gain1 : Gain  Gain=sb
  Gain2 : Gain  Gain=sf
  Gain3 : Gain  Gain=sf
  Integrator : Integrator  InitialCondition=u0
  Integrator1 : Integrator  InitialCondition=v0
  MATLAB Function : MATLAB Function  TreatAsAtomicUnit=on
  MATLAB Function1 : MATLAB Function  TreatAsAtomicUnit=on
  Product{,1..3} (4 alike) : Product
  Scope : Scope
  Sum{,1..3} (4 alike) : Sum  Inputs=|+-
  w1 : Gain  Gain=w
  w2 : Gain  Gain=-w
  u_i : Outport
  v_i : Outport  Port=2
  wires:
  Product2/1 -> Add/3
  Gain3/1 -> Product3/1
  w2/1 -> Add1/1
  Discrete Impulse1/1 -> Gain1/1
  Gain1/1 -> Product1/1
  Discrete Impulse/1 -> Gain/1
  Constant/1 -> MATLAB Function/2(k)
  Sum2/1 -> Product/2
  Add1/1 -> Integrator1/1
  Product1/1 -> Add1/3, Scope/1
  MATLAB Function/1(y) -> Add/1
  Discrete Impulse3/1 -> Gain3/1
  Product/1 -> Add/2
  Sum3/1 -> Product1/2
  Constant1/1 -> MATLAB Function1/2(k)
  w1/1 -> Add/4
  Integrator1/1 -> v_i/1, Sum3/2, Sum1/2, MATLAB Function1/3(x), w1/1
  Gain/1 -> Product/1
  Constant3/1 -> MATLAB Function1/1(r)
  Add/1 -> Integrator/1
  v_i+1/1 -> Sum1/1
  Sum/1 -> Product2/2
  Gain2/1 -> Product2/1
  Discrete Impulse2/1 -> Gain2/1
  Product3/1 -> Add1/2
  MATLAB Function1/1(y) -> Add1/4
  Constant2/1 -> MATLAB Function/3(r)
  u_i+1/1 -> Sum/1
  Sum1/1 -> Product3/2
  Integrator/1 -> u_i/1, Sum2/2, Sum/2, MATLAB Function/1(x), w2/1
  u_i-1/1 -> Sum2/1
  v_i-1/1 -> Sum3/1

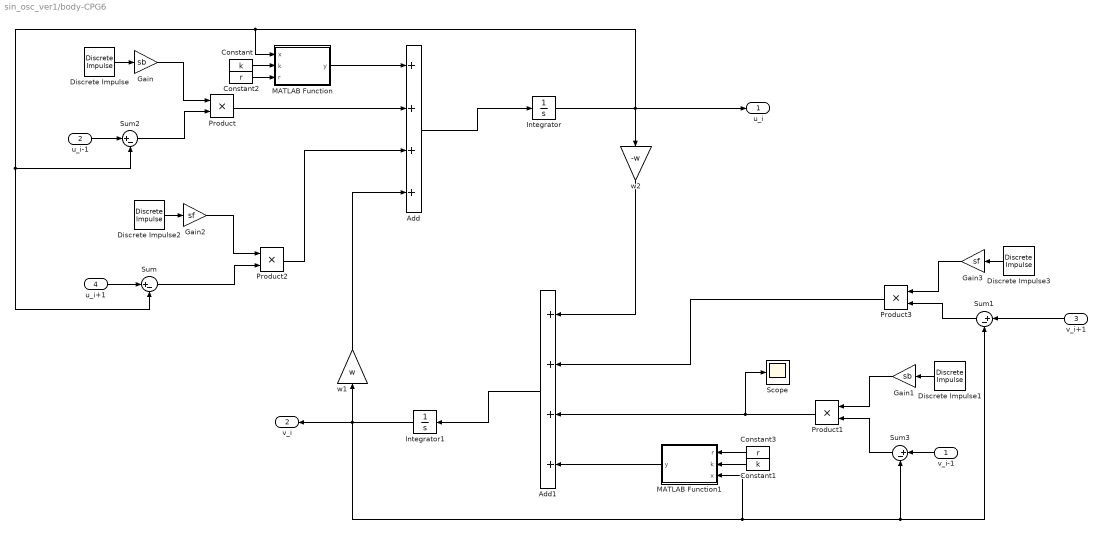
== system sin_osc_ver1/body-CPG6 ==
  v_i-1 : Inport
  u_i-1 : Inport  Port=2
  v_i+1 : Inport  Port=3
  u_i+1 : Inport  Port=4
  Add : Sum  Inputs=++++
  Add1 : Sum  Inputs=++++
  Constant : Constant  Value=k
  Constant1 : Constant  Value=k
  Constant2 : Constant  Value=r
  Constant3 : Constant  Value=r
  Discrete Impulse : dspsrcs4/Discrete  Impulse  Delay=round(6*deltaT/t_sample)+1  SampleTime=t_sample  FrameSample=1  OutputFrames=off  dataType=double  isSigned=on  wordLen=16  udDataType=sfix(16)  fracBitsMode=Best precision  numFracBits=15  OutDataTypeStr=double  LastOutDataTypeStr=double
  Discrete Impulse1 : dspsrcs4/Discrete  Impulse  Delay=round(6*deltaT/t_sample)  SampleTime=t_sample  FrameSample=1  OutputFrames=off  dataType=double  isSigned=on  wordLen=16  udDataType=sfix(16)  fracBitsMode=Best precision  numFracBits=15  OutDataTypeStr=double  LastOutDataTypeStr=double
  Discrete Impulse2 : dspsrcs4/Discrete  Impulse  Delay=round(6*deltaT/t_sample)+1  SampleTime=t_sample  FrameSample=1  OutputFrames=off  dataType=double  isSigned=on  wordLen=16  udDataType=sfix(16)  fracBitsMode=Best precision  numFracBits=15  OutDataTypeStr=double  LastOutDataTypeStr=double
  Discrete Impulse3 : dspsrcs4/Discrete  Impulse  Delay=round(6*deltaT/t_sample)  SampleTime=t_sample  FrameSample=1  OutputFrames=off  dataType=double  isSigned=on  wordLen=16  udDataType=sfix(16)  fracBitsMode=Best precision  numFracBits=15  OutDataTypeStr=double  LastOutDataTypeStr=double
  Gain : Gain  Gain=sb
  Gain1 : Gain  Gain=sb
  Gain2 : Gain  Gain=sf
  Gain3 : Gain  Gain=sf
  Integrator : Integrator  InitialCondition=u0
  Integrator1 : Integrator  InitialCondition=v0
  MATLAB Function : MATLAB Function  TreatAsAtomicUnit=on
  MATLAB Function1 : MATLAB Function  TreatAsAtomicUnit=on
  Product{,1..3} (4 alike) : Product
  Scope : Scope
  Sum{,1..3} (4 alike) : Sum  Inputs=|+-
  w1 : Gain  Gain=w
  w2 : Gain  Gain=-w
  u_i : Outport
  v_i : Outport  Port=2
  wires:
  Product2/1 -> Add/3
  Gain3/1 -> Product3/1
  w2/1 -> Add1/1
  Discrete Impulse1/1 -> Gain1/1
  Gain1/1 -> Product1/1
  Discrete Impulse/1 -> Gain/1
  Constant/1 -> MATLAB Function/2(k)
  Sum2/1 -> Product/2
  Add1/1 -> Integrator1/1
  Product1/1 -> Add1/3, Scope/1
  MATLAB Function/1(y) -> Add/1
  Discrete Impulse3/1 -> Gain3/1
  Product/1 -> Add/2
  Sum3/1 -> Product1/2
  Constant1/1 -> MATLAB Function1/2(k)
  w1/1 -> Add/4
  Integrator1/1 -> v_i/1, Sum3/2, Sum1/2, MATLAB Function1/3(x), w1/1
  Gain/1 -> Product/1
  Constant3/1 -> MATLAB Function1/1(r)
  Add/1 -> Integrator/1
  v_i+1/1 -> Sum1/1
  Sum/1 -> Product2/2
  Gain2/1 -> Product2/1
  Discrete Impulse2/1 -> Gain2/1
  Product3/1 -> Add1/2
  MATLAB Function1/1(y) -> Add1/4
  Constant2/1 -> MATLAB Function/3(r)
  u_i+1/1 -> Sum/1
  Sum1/1 -> Product3/2
  Integrator/1 -> u_i/1, Sum2/2, Sum/2, MATLAB Function/1(x), w2/1
  u_i-1/1 -> Sum2/1
  v_i-1/1 -> Sum3/1

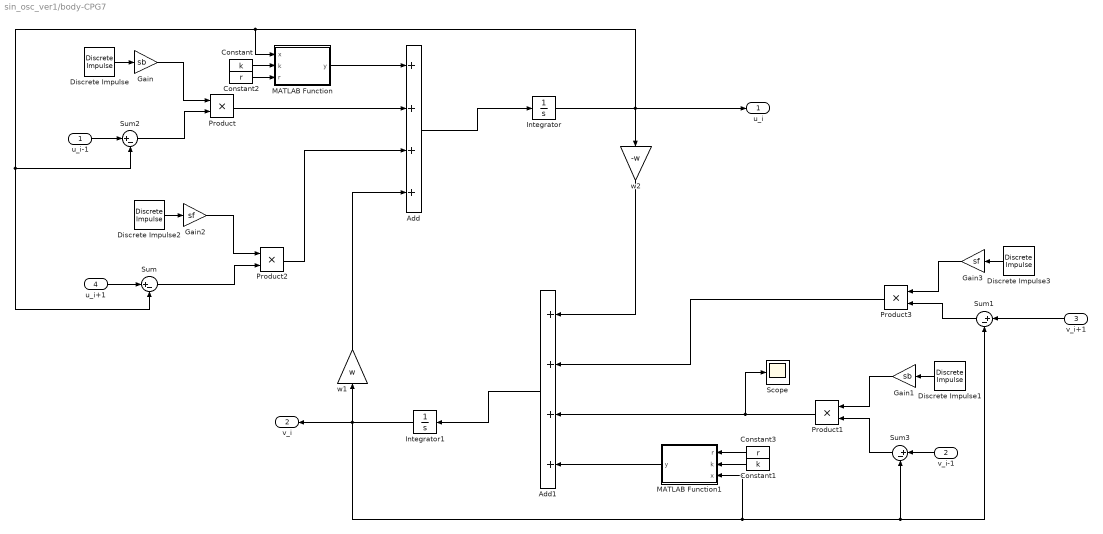
== system sin_osc_ver1/body-CPG7 ==
  u_i-1 : Inport
  v_i-1 : Inport  Port=2
  v_i+1 : Inport  Port=3
  u_i+1 : Inport  Port=4
  Add : Sum  Inputs=++++
  Add1 : Sum  Inputs=++++
  Constant : Constant  Value=k
  Constant1 : Constant  Value=k
  Constant2 : Constant  Value=r
  Constant3 : Constant  Value=r
  Discrete Impulse : dspsrcs4/Discrete  Impulse  Delay=round(7*deltaT/t_sample)+1  SampleTime=t_sample  FrameSample=1  OutputFrames=off  dataType=double  isSigned=on  wordLen=16  udDataType=sfix(16)  fracBitsMode=Best precision  numFracBits=15  OutDataTypeStr=double  LastOutDataTypeStr=double
  Discrete Impulse1 : dspsrcs4/Discrete  Impulse  Delay=round(7*deltaT/t_sample)  SampleTime=t_sample  FrameSample=1  OutputFrames=off  dataType=double  isSigned=on  wordLen=16  udDataType=sfix(16)  fracBitsMode=Best precision  numFracBits=15  OutDataTypeStr=double  LastOutDataTypeStr=double
  Discrete Impulse2 : dspsrcs4/Discrete  Impulse  Delay=round(7*deltaT/t_sample)+1  SampleTime=t_sample  FrameSample=1  OutputFrames=off  dataType=double  isSigned=on  wordLen=16  udDataType=sfix(16)  fracBitsMode=Best precision  numFracBits=15  OutDataTypeStr=double  LastOutDataTypeStr=double
  Discrete Impulse3 : dspsrcs4/Discrete  Impulse  Delay=round(7*deltaT/t_sample)  SampleTime=t_sample  FrameSample=1  OutputFrames=off  dataType=double  isSigned=on  wordLen=16  udDataType=sfix(16)  fracBitsMode=Best precision  numFracBits=15  OutDataTypeStr=double  LastOutDataTypeStr=double
  Gain : Gain  Gain=sb
  Gain1 : Gain  Gain=sb
  Gain2 : Gain  Gain=sf
  Gain3 : Gain  Gain=sf
  Integrator : Integrator  InitialCondition=u0
  Integrator1 : Integrator  InitialCondition=v0
  MATLAB Function : MATLAB Function  TreatAsAtomicUnit=on
  MATLAB Function1 : MATLAB Function  TreatAsAtomicUnit=on
  Product{,1..3} (4 alike) : Product
  Scope : Scope
  Sum{,1..3} (4 alike) : Sum  Inputs=|+-
  w1 : Gain  Gain=w
  w2 : Gain  Gain=-w
  u_i : Outport
  v_i : Outport  Port=2
  wires:
  Product2/1 -> Add/3
  Gain3/1 -> Product3/1
  w2/1 -> Add1/1
  Discrete Impulse1/1 -> Gain1/1
  Gain1/1 -> Product1/1
  Discrete Impulse/1 -> Gain/1
  Constant/1 -> MATLAB Function/2(k)
  Sum2/1 -> Product/2
  Add1/1 -> Integrator1/1
  Product1/1 -> Add1/3, Scope/1
  MATLAB Function/1(y) -> Add/1
  Discrete Impulse3/1 -> Gain3/1
  Product/1 -> Add/2
  Sum3/1 -> Product1/2
  Constant1/1 -> MATLAB Function1/2(k)
  w1/1 -> Add/4
  Integrator1/1 -> v_i/1, Sum3/2, Sum1/2, MATLAB Function1/3(x), w1/1
  Gain/1 -> Product/1
  Constant3/1 -> MATLAB Function1/1(r)
  Add/1 -> Integrator/1
  v_i+1/1 -> Sum1/1
  Sum/1 -> Product2/2
  Gain2/1 -> Product2/1
  Discrete Impulse2/1 -> Gain2/1
  Product3/1 -> Add1/2
  MATLAB Function1/1(y) -> Add1/4
  Constant2/1 -> MATLAB Function/3(r)
  u_i+1/1 -> Sum/1
  Sum1/1 -> Product3/2
  Integrator/1 -> u_i/1, Sum2/2, Sum/2, MATLAB Function/1(x), w2/1
  u_i-1/1 -> Sum2/1
  v_i-1/1 -> Sum3/1

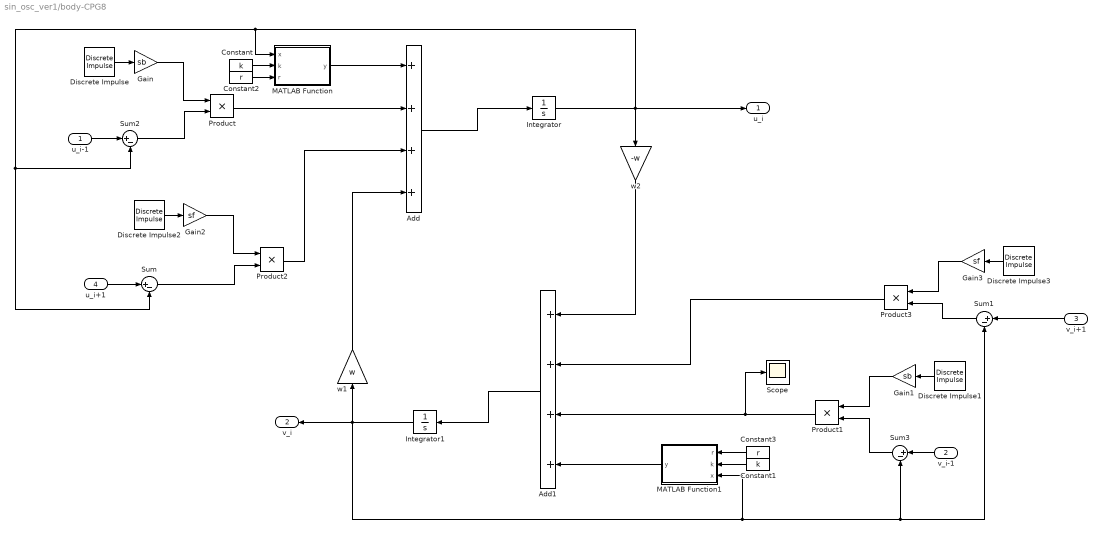
== system sin_osc_ver1/body-CPG8 ==
  u_i-1 : Inport
  v_i-1 : Inport  Port=2
  v_i+1 : Inport  Port=3
  u_i+1 : Inport  Port=4
  Add : Sum  Inputs=++++
  Add1 : Sum  Inputs=++++
  Constant : Constant  Value=k
  Constant1 : Constant  Value=k
  Constant2 : Constant  Value=r
  Constant3 : Constant  Value=r
  Discrete Impulse : dspsrcs4/Discrete  Impulse  Delay=round(8*deltaT/t_sample)+1  SampleTime=t_sample  FrameSample=1  OutputFrames=off  dataType=double  isSigned=on  wordLen=16  udDataType=sfix(16)  fracBitsMode=Best precision  numFracBits=15  OutDataTypeStr=double  LastOutDataTypeStr=double
  Discrete Impulse1 : dspsrcs4/Discrete  Impulse  Delay=round(8*deltaT/t_sample)  SampleTime=t_sample  FrameSample=1  OutputFrames=off  dataType=double  isSigned=on  wordLen=16  udDataType=sfix(16)  fracBitsMode=Best precision  numFracBits=15  OutDataTypeStr=double  LastOutDataTypeStr=double
  Discrete Impulse2 : dspsrcs4/Discrete  Impulse  Delay=round(8*deltaT/t_sample)+1  SampleTime=t_sample  FrameSample=1  OutputFrames=off  dataType=double  isSigned=on  wordLen=16  udDataType=sfix(16)  fracBitsMode=Best precision  numFracBits=15  OutDataTypeStr=double  LastOutDataTypeStr=double
  Discrete Impulse3 : dspsrcs4/Discrete  Impulse  Delay=round(8*deltaT/t_sample)  SampleTime=t_sample  FrameSample=1  OutputFrames=off  dataType=double  isSigned=on  wordLen=16  udDataType=sfix(16)  fracBitsMode=Best precision  numFracBits=15  OutDataTypeStr=double  LastOutDataTypeStr=double
  Gain : Gain  Gain=sb
  Gain1 : Gain  Gain=sb
  Gain2 : Gain  Gain=sf
  Gain3 : Gain  Gain=sf
  Integrator : Integrator  InitialCondition=u0
  Integrator1 : Integrator  InitialCondition=v0
  MATLAB Function : MATLAB Function  TreatAsAtomicUnit=on
  MATLAB Function1 : MATLAB Function  TreatAsAtomicUnit=on
  Product{,1..3} (4 alike) : Product
  Scope : Scope
  Sum{,1..3} (4 alike) : Sum  Inputs=|+-
  w1 : Gain  Gain=w
  w2 : Gain  Gain=-w
  u_i : Outport
  v_i : Outport  Port=2
  wires:
  Product2/1 -> Add/3
  Gain3/1 -> Product3/1
  w2/1 -> Add1/1
  Discrete Impulse1/1 -> Gain1/1
  Gain1/1 -> Product1/1
  Discrete Impulse/1 -> Gain/1
  Constant/1 -> MATLAB Function/2(k)
  Sum2/1 -> Product/2
  Add1/1 -> Integrator1/1
  Product1/1 -> Add1/3, Scope/1
  MATLAB Function/1(y) -> Add/1
  Discrete Impulse3/1 -> Gain3/1
  Product/1 -> Add/2
  Sum3/1 -> Product1/2
  Constant1/1 -> MATLAB Function1/2(k)
  w1/1 -> Add/4
  Integrator1/1 -> v_i/1, Sum3/2, Sum1/2, MATLAB Function1/3(x), w1/1
  Gain/1 -> Product/1
  Constant3/1 -> MATLAB Function1/1(r)
  Add/1 -> Integrator/1
  v_i+1/1 -> Sum1/1
  Sum/1 -> Product2/2
  Gain2/1 -> Product2/1
  Discrete Impulse2/1 -> Gain2/1
  Product3/1 -> Add1/2
  MATLAB Function1/1(y) -> Add1/4
  Constant2/1 -> MATLAB Function/3(r)
  u_i+1/1 -> Sum/1
  Sum1/1 -> Product3/2
  Integrator/1 -> u_i/1, Sum2/2, Sum/2, MATLAB Function/1(x), w2/1
  u_i-1/1 -> Sum2/1
  v_i-1/1 -> Sum3/1

== system sin_osc_ver1/body-CPG9 ==
  u_i-1 : Inport
  v_i-1 : Inport  Port=2
  v_i+1 : Inport  Port=3
  u_i+1 : Inport  Port=4
  Add : Sum  Inputs=++++
  Add1 : Sum  Inputs=++++
  Constant : Constant  Value=k
  Constant1 : Constant  Value=k
  Constant2 : Constant  Value=r
  Constant3 : Constant  Value=r
  Discrete Impulse : dspsrcs4/Discrete  Impulse  Delay=round(9*deltaT/t_sample)+1  SampleTime=t_sample  FrameSample=1  OutputFrames=off  dataType=double  isSigned=on  wordLen=16  udDataType=sfix(16)  fracBitsMode=Best precision  numFracBits=15  OutDataTypeStr=double  LastOutDataTypeStr=double
  Discrete Impulse1 : dspsrcs4/Discrete  Impulse  Delay=round(9*deltaT/t_sample)  SampleTime=t_sample  FrameSample=1  OutputFrames=off  dataType=double  isSigned=on  wordLen=16  udDataType=sfix(16)  fracBitsMode=Best precision  numFracBits=15  OutDataTypeStr=double  LastOutDataTypeStr=double
  Discrete Impulse2 : dspsrcs4/Discrete  Impulse  Delay=round(9*deltaT/t_sample)+1  SampleTime=t_sample  FrameSample=1  OutputFrames=off  dataType=double  isSigned=on  wordLen=16  udDataType=sfix(16)  fracBitsMode=Best precision  numFracBits=15  OutDataTypeStr=double  LastOutDataTypeStr=double
  Discrete Impulse3 : dspsrcs4/Discrete  Impulse  Delay=round(9*deltaT/t_sample)  SampleTime=t_sample  FrameSample=1  OutputFrames=off  dataType=double  isSigned=on  wordLen=16  udDataType=sfix(16)  fracBitsMode=Best precision  numFracBits=15  OutDataTypeStr=double  LastOutDataTypeStr=double
  Gain : Gain  Gain=sb
  Gain1 : Gain  Gain=sb
  Gain2 : Gain  Gain=sf
  Gain3 : Gain  Gain=sf
  Integrator : Integrator  InitialCondition=u0
  Integrator1 : Integrator  InitialCondition=v0
  MATLAB Function : MATLAB Function  TreatAsAtomicUnit=on
  MATLAB Function1 : MATLAB Function  TreatAsAtomicUnit=on
  Product{,1..3} (4 alike) : Product
  Scope : Scope
  Sum{,1..3} (4 alike) : Sum  Inputs=|+-
  w1 : Gain  Gain=w
  w2 : Gain  Gain=-w
  u_i : Outport
  v_i : Outport  Port=2
  wires:
  Product2/1 -> Add/3
  Gain3/1 -> Product3/1
  w2/1 -> Add1/1
  Discrete Impulse1/1 -> Gain1/1
  Gain1/1 -> Product1/1
  Discrete Impulse/1 -> Gain/1
  Constant/1 -> MATLAB Function/2(k)
  Sum2/1 -> Product/2
  Add1/1 -> Integrator1/1
  Product1/1 -> Add1/3, Scope/1
  MATLAB Function/1(y) -> Add/1
  Discrete Impulse3/1 -> Gain3/1
  Product/1 -> Add/2
  Sum3/1 -> Product1/2
  Constant1/1 -> MATLAB Function1/2(k)
  w1/1 -> Add/4
  Integrator1/1 -> v_i/1, Sum3/2, Sum1/2, MATLAB Function1/3(x), w1/1
  Gain/1 -> Product/1
  Constant3/1 -> MATLAB Function1/1(r)
  Add/1 -> Integrator/1
  v_i+1/1 -> Sum1/1
  Sum/1 -> Product2/2
  Gain2/1 -> Product2/1
  Discrete Impulse2/1 -> Gain2/1
  Product3/1 -> Add1/2
  MATLAB Function1/1(y) -> Add1/4
  Constant2/1 -> MATLAB Function/3(r)
  u_i+1/1 -> Sum/1
  Sum1/1 -> Product3/2
  Integrator/1 -> u_i/1, Sum2/2, Sum/2, MATLAB Function/1(x), w2/1
  u_i-1/1 -> Sum2/1
  v_i-1/1 -> Sum3/1
